simulink model "powerwindow"  (Simulink 6.0)
settings: Solver=FixedStepDiscrete  StartTime=0.0  StopTime=inf  FixedStep=1e-4  RelTol=1e-3
libraries: simulink x6
settings Model: Creator=The MathWorks Inc.  LastModifiedBy=batserve  ExtModeAutoUpdateStatusClock=off  ProdHWDeviceType=Specified
settings DataIOCC: SignalLoggingName=sigsOut
settings OptimizationCC: BooleanDataType=off
settings DebuggingCC: CheckExecutionContextPreStartOutputMsg=on  CheckExecutionContextRuntimeOutputMsg=on  SolverPrmCheckMsg=none
settings HardwareCC: ProdBitPerShort=32  ProdBitPerInt=16  ProdHWDeviceType=Specified  TargetUnknown=on

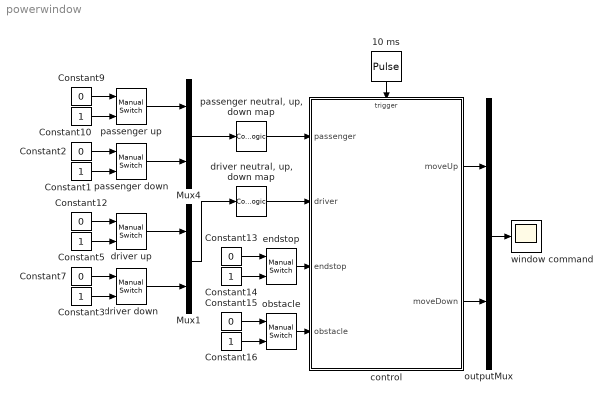
== system powerwindow ==
  10 ms : DiscretePulseGenerator  Orientation=down  PulseType=Time based  Period=1e-2  PulseWidth=50  SampleTime=1e-3
  Constant{1,3,5,10,14,16} (6 alike) : Constant
  Constant{2,7,9,12..13,15} (6 alike) : Constant  Value=0
  Mux1 : Mux  Inputs=2
  Mux4 : Mux  Inputs=2
  control : Stateflow chart  TreatAsAtomicUnit=on  PropExecContextAcrossSSBoundary=on
  "driver neutral, up, down map" : CombinatorialLogic  TruthTable=[1 0 0;0 0 1;0 1 0;1 0 0]
  driver down : simulink/Signal Routing/Manual Switch  sw=1  action=0
  driver up : simulink/Signal Routing/Manual Switch  sw=1  action=0
  endstop : simulink/Signal Routing/Manual Switch  sw=1  action=0
  obstacle : simulink/Signal Routing/Manual Switch  sw=1  action=0
  outputMux : Mux  Inputs=2
  "passenger neutral, up, down map" : CombinatorialLogic  TruthTable=[1 0 0;0 0 1;0 1 0;1 0 0]
  passenger down : simulink/Signal Routing/Manual Switch  sw=1  action=0
  passenger up : simulink/Signal Routing/Manual Switch  sw=1  action=0
  window command : Scope
      settings: YMin=0  YMax=1
  wires:
  Constant9/1 -> passenger up/1
  Constant10/1 -> passenger up/2
  Constant2/1 -> passenger down/1
  Constant1/1 -> passenger down/2
  10 ms/1 -> control/Trigger
  passenger down/1 -> Mux4/2
  Constant12/1 -> driver up/1
  Constant5/1 -> driver up/2
  Constant7/1 -> driver down/1
  Constant3/1 -> driver down/2
  driver down/1 -> Mux1/2
  Mux4/1 -> "passenger neutral, up, down map"/1
  Mux1/1 -> "driver neutral, up, down map"/1
  "passenger neutral, up, down map"/1 -> control/1(passenger)
  "driver neutral, up, down map"/1 -> control/2(driver)
  passenger up/1 -> Mux4/1
  driver up/1 -> Mux1/1
  control/1(moveUp) -> outputMux/1
  control/2(moveDown) -> outputMux/2
  outputMux/1 -> window command/1
  Constant13/1 -> endstop/1
  Constant14/1 -> endstop/2
  Constant15/1 -> obstacle/1
  Constant16/1 -> obstacle/2
  endstop/1 -> control/3(endstop)
  obstacle/1 -> control/4(obstacle)

== stateflow chart control ==
  settings: executeAtInitialization=1
  state emergencyDown
    entry:
    moveUp = 0;
    moveDown = 1;
  state safe
    state driverUp
      entry: moveUp = 1;
      exit: moveUp = 0;
      state iniDriverUp
      state DriverUp
      state autoDriverUp
      iniDriverUp -> (junction 26) : after(100,ticks)
      (junction 26) -> DriverUp
      (junction 26) -> autoDriverUp : [driver[1]]
    state driverDown
      entry: moveDown = 1;
      exit: moveDown = 0;
      state iniDriverDown
      state DriverDown
      state autoDriverDown
      iniDriverDown -> (junction 25) : after(100,ticks)
      (junction 25) -> autoDriverDown : [driver[1]]
      (junction 25) -> DriverDown
    state driverNeutral
      entry:
      moveUp = 0;
      moveDown = 0;
      state passengerneutral
        entry:
        moveUp = 0;
        moveDown = 0;
      state passengerUp
        entry: moveUp = 1;
        exit: moveUp = 0;
        state iniPassengerUp
        state PassengerUp
        state autoPassengerUp
        (junction 24) -> PassengerUp
        (junction 24) -> autoPassengerUp : [passenger[1]]
        iniPassengerUp -> (junction 24) : after(100,ticks)
      state passengerDown
        entry: moveDown = 1;
        exit: moveDown = 0;
        state iniPassengerDown
        state passengerDown
        state autoPassengerDown
        (junction 23) -> autoPassengerDown : [passenger[1]]
        iniPassengerDown -> (junction 23) : after(100,ticks)
        (junction 23) -> safe.driverNeutral.passengerDown.passengerDown
      safe.driverNeutral.passengerDown.passengerDown -> passengerneutral : [passenger[1]]
      safe.driverNeutral.passengerDown -> passengerneutral : [endstop]
      PassengerUp -> passengerneutral : [passenger[1]]
      passengerUp -> passengerneutral : [endstop]
      passengerneutral -> iniPassengerDown : [passenger[3]]
      passengerneutral -> iniPassengerUp : [passenger[2]]
      safe.driverNeutral.passengerDown -> PassengerUp : [passenger[2]]
      passengerUp -> safe.driverNeutral.passengerDown.passengerDown : [passenger[3]]
      (default) -> passengerneutral
    driverNeutral -> iniDriverDown : [driver[3]]
    driverUp -> DriverDown : [driver[3]]
    driverDown -> DriverUp : [driver[2]]
    driverNeutral -> iniDriverUp : [driver[2]]
    DriverDown -> driverNeutral : [driver[1]]
    DriverUp -> driverNeutral : [driver[1]]
    driverDown -> driverNeutral : [endstop]
    driverUp -> driverNeutral : [endstop]
    (default) -> driverNeutral
  emergencyDown -> passengerneutral : [endstop | after(100,ticks)]
  safe -> emergencyDown : [obstacle]
  (default) -> safe
  data: passenger input boolean size=3; driver input boolean size=3; moveUp output double; moveDown output double; endstop input double; obstacle input double
  events: ticks input RISING_EDGE_EVENT
